simulink model "LQR_FNM"  (R2014a)
settings: Solver=ode45  StartTime=0.0  StopTime=6000  RelTol=1e-3
settings Model: Creator=Imaculada  LastModifiedBy=Imaculada

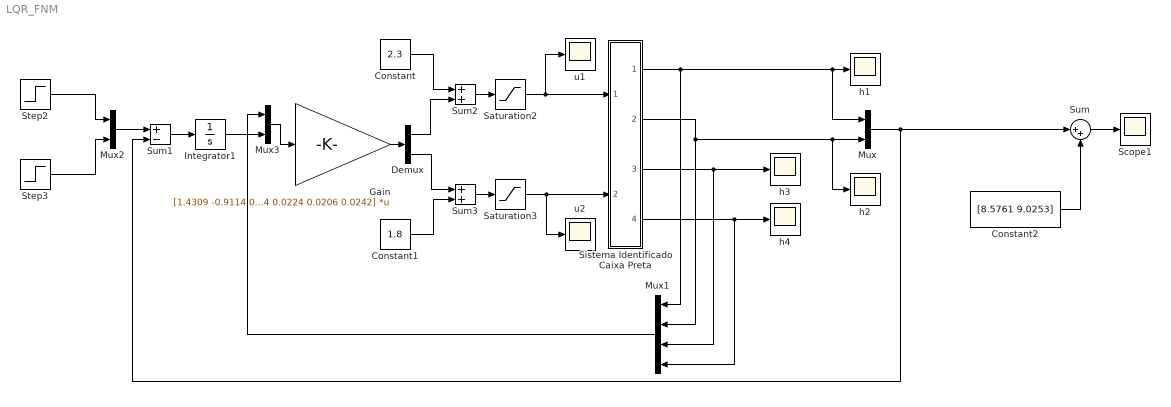
== system LQR_FNM ==
  Constant : Constant  Value=2.3
  Constant1 : Constant  Value=1.8
  Constant2 : Constant  Value=[8.5761 9.0253]
  Demux : Demux  Outputs=2
  Gain : Gain  Gain=[1.4309 -0.9114 0.2026 -0.3160 -0.0152 0.0145 ; -1.3015 -0.1473 -0.1544 0.0224 0.0206 0.0242]  Multiplication=Matrix(K*u)
  Integrator1 : Integrator
  Mux : Mux  Inputs=2
  Mux1 : Mux
  Mux2 : Mux  Inputs=2
  Mux3 : Mux  Inputs=2
  Saturation2 : Saturate  UpperLimit=1.5  LowerLimit=-1.5
  Saturation3 : Saturate  UpperLimit=1.5  LowerLimit=-1.5
  Scope1 : Scope
      settings: SaveName=Simulado  SampleInput=on  SampleTime=10^-1
  Sistema Identificado Caixa Preta : Subsystem
  Step2 : Step  Time=2300  SampleTime=0
  Step3 : Step  Time=3100  SampleTime=0
  Sum : Sum  Inputs=|++
  Sum1 : Sum  Inputs=+-
  Sum2 : Sum
  Sum3 : Sum
  h{1..4} (4 alike) : Scope
      h1 settings: YMin=9  YMax=17.5  SaveName=ScopeData4
      h2 settings: TimeRange=6000  SaveName=ScopeData5
      h3 settings: SaveName=ScopeData3
      h4 settings: SaveName=ScopeData6
  u1 : Scope
      settings: SaveName=ScopeData2
  u2 : Scope
  wires:
  Gain/1 -> Demux/1
  Sistema Identificado Caixa Preta/3(h3) -> Mux1/3, h3/1
  Sistema Identificado Caixa Preta/4(h4) -> Mux1/4, h4/1
  Mux/1 -> Sum/1, Sum1/2
  Mux2/1 -> Sum1/1
  Mux3/1 -> Gain/1
  Sum1/1 -> Integrator1/1
  Mux1/1 -> Mux3/1
  Demux/1 -> Sum2/2
  Step3/1 -> Mux2/2
  Step2/1 -> Mux2/1
  Integrator1/1 -> Mux3/2
  Demux/2 -> Sum3/1
  Sistema Identificado Caixa Preta/1(h1) -> h1/1, Mux/1, Mux1/1
  Sistema Identificado Caixa Preta/2(h2) -> h2/1, Mux/2, Mux1/2
  Constant1/1 -> Sum3/2
  Constant/1 -> Sum2/1
  Sum2/1 -> Saturation2/1
  Sum3/1 -> Saturation3/1
  Saturation2/1 -> Sistema Identificado Caixa Preta/1(u1), u1/1
  Saturation3/1 -> Sistema Identificado Caixa Preta/2(u2), u2/1
  Sum/1 -> Scope1/1
  Constant2/1 -> Sum/2

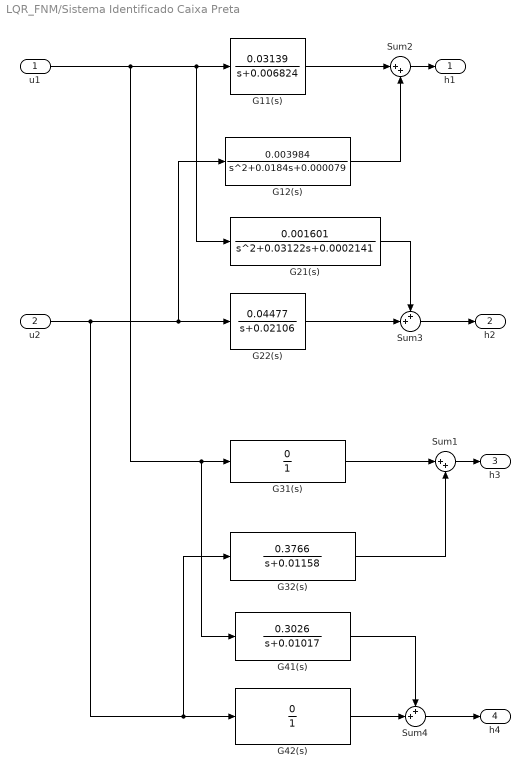
== system LQR_FNM/Sistema Identificado Caixa Preta ==
  u1 : Inport
  u2 : Inport  Port=2
  G11(s) : TransferFcn  Numerator=[0 0.03139]  Denominator=[1 0.006824]
  G12(s) : TransferFcn  Numerator=[0 0 0.003984]  Denominator=[1 0.0184 0.000079]
  G21(s) : TransferFcn  Numerator=[0 0 0.001601]  Denominator=[1 0.03122 0.0002141]
  G22(s) : TransferFcn  Numerator=[0 0.04477]  Denominator=[1 0.02106]
  G31(s) : TransferFcn  Numerator=0  Denominator=1
  G32(s) : TransferFcn  Numerator=[0 0.3766]  Denominator=[1 0.01158]
  G41(s) : TransferFcn  Numerator=[0.3026]  Denominator=[1 0.01017]
  G42(s) : TransferFcn  Numerator=0  Denominator=1
  Sum1 : Sum  Inputs=|++
  Sum2 : Sum  Inputs=|++
  Sum3 : Sum  Inputs=++|
  Sum4 : Sum  Inputs=++|
  h1 : Outport
  h2 : Outport  Port=2
  h3 : Outport  Port=3
  h4 : Outport  Port=4
  wires:
  G11(s)/1 -> Sum2/1
  G22(s)/1 -> Sum3/2
  G12(s)/1 -> Sum2/2
  G21(s)/1 -> Sum3/1
  Sum2/1 -> h1/1
  Sum3/1 -> h2/1
  u1/1 -> G41(s)/1, G31(s)/1, G21(s)/1, G11(s)/1
  u2/1 -> G32(s)/1, G42(s)/1, G22(s)/1, G12(s)/1
  G31(s)/1 -> Sum1/1
  G42(s)/1 -> Sum4/2
  G32(s)/1 -> Sum1/2
  G41(s)/1 -> Sum4/1
  Sum1/1 -> h3/1
  Sum4/1 -> h4/1
